simulink model "Target_Control_System"  (R2021b)
settings: Solver=FixedStepDiscrete  StartTime=0.0  StopTime=5  RelTol=1e-3
PreLoadFcn:
  | RTWConfigurationCB('preloadfcn', bdroot);
PostLoadFcn:
  | load('configuration/data_struct.mat');
  | load('configuration/fluxMaps_propMotor.mat');
  | load('configuration/parameterInit_PROP.mat');
  | load('configuration/parameterInit_PUMP.mat');
  | load('configuration/parameterInit_PITCH.mat');
  | load('configuration/parameterInit_TILT.mat');
  | %load('configuration/base_workspace_signal_definition.mat');
  | %load('resolvedatastores_to_baseworkspace_for_faster_simulation.mat');
model workspace (MAT data in the model file):
  SIMULATION_OPTIONS : Simulink.Parameter (value not decoded)
  TARGET_CODE_GEN : Simulink.Parameter (value not decoded)
  TCS_SAMPLE_FREQ_HZ : Simulink.Parameter (value not decoded)
symbols that are objects in the model workspace (value not decoded): TARGET_CODE_GEN, TCS_SAMPLE_FREQ_HZ
undefined symbols (not defined in the file): A_DQ_REF_LPF_INIT__PITCH, A_DQ_REF_LPF_INIT__PROP, A_DQ_REF_LPF_INIT__PUMP, A_DQ_REF_LPF_INIT__TILT, A_OBSERVER_CONFIDENCE_INIT__PITCH, A_OBSERVER_CONFIDENCE_INIT__PROP, A_OBSERVER_CONFIDENCE_INIT__PUMP, A_OBSERVER_CONFIDENCE_INIT__TILT, ACTUATOR_MAX_ANGLE_TRIP__PITCH, ACTUATOR_MIN_ANGLE_TRIP__PITCH, ACTUATOR_POS_SENSOR_INV_DIRECTION__PITCH, ACTUATOR_POS_SENSOR_INV_DIRECTION__TILT, ACTUATOR_POS_SENSOR_OFFSET__PITCH, ACTUATOR_POS_SENSOR_OFFSET__TILT, ADC_scaler1_baseaddr_TILT, ADC_SCALER_FLOAT_TO_FIXPOINT_EXPANSION, ANGLE_ELEC_FROM_SENSOR_OFFSET_INIT__PITCH, ANGLE_ELEC_FROM_SENSOR_OFFSET_INIT__PROP, ANGLE_ELEC_FROM_SENSOR_OFFSET_INIT__PUMP, ANGLE_ELEC_FROM_SENSOR_OFFSET_INIT__TILT, AUTO_CLEAR_FAULTS_ENABLED__PITCH, AUTO_CLEAR_FAULTS_ENABLED__PROP, AUTO_CLEAR_FAULTS_ENABLED__PUMP, AUTO_CLEAR_FAULTS_ENABLED__TILT, AUTO_CLEAR_FAULTS_WAIT_TICKS__PITCH, AUTO_CLEAR_FAULTS_WAIT_TICKS__PROP, AUTO_CLEAR_FAULTS_WAIT_TICKS__PUMP, AUTO_CLEAR_FAULTS_WAIT_TICKS__TILT, AUTO_I_ZERO_IDLE_TICKS__PITCH, AUTO_I_ZERO_IDLE_TICKS__PROP, AUTO_I_ZERO_IDLE_TICKS__PUMP, AUTO_I_ZERO_IDLE_TICKS__TILT, AUTO_I_ZERO_OFFSET_IDC_THRESHOLD__PITCH, AUTO_I_ZERO_OFFSET_IDC_THRESHOLD__PROP, AUTO_I_ZERO_OFFSET_IDC_THRESHOLD__PUMP, AUTO_I_ZERO_OFFSET_IDC_THRESHOLD__TILT, AUTO_I_ZERO_OFFSET_IPH_THRESHOLD__PITCH, AUTO_I_ZERO_OFFSET_IPH_THRESHOLD__PROP, AUTO_I_ZERO_OFFSET_IPH_THRESHOLD__PUMP, AUTO_I_ZERO_OFFSET_IPH_THRESHOLD__TILT, AUTO_SENSORLESS_SWITCHOVER_DISABLE_OMEGA, AUTO_SENSORLESS_SWITCHOVER_ENABLE_OMEGA, AUTO_SENSORLESS_SWITCHOVER_MIN_CONFIDENCE, AUXILIARY_PROTECTION_UNIT_BASEADDR__TILT, blanking_max_error_omega_INIT_PITCH, blanking_max_error_omega_INIT_TILT, blanking_max_error_position_INIT_PITCH, blanking_max_error_position_INIT_TILT, BRUTE_START_I_Q_REF_RAMP_SPEED__PITCH, BRUTE_START_I_Q_REF_RAMP_SPEED__PROP, BRUTE_START_I_Q_REF_RAMP_SPEED__PUMP, BRUTE_START_I_Q_REF_RAMP_SPEED__TILT, CONTROL_LOOP_DT_INIT__PITCH, CONTROL_LOOP_DT_INIT__PROP, CONTROL_LOOP_DT_INIT__PUMP, CONTROL_LOOP_DT_INIT__TILT, CORRECTION_FILTER_SCALE__PITCH, CORRECTION_FILTER_SCALE__PROP, CORRECTION_FILTER_SCALE__PUMP, CORRECTION_FILTER_SCALE__TILT ... (+458)
libraries: simulink x178, Reusables_Lib x24
(part 27 of 47)

== system Target_Control_System/Target_Control_System/InterruptFunction/tiltMotor_isrTask/pwmGeneration/Subsystem/Calculate Duty Cycles ==
  fUaRef : Inport
  fUbRef : Inport  Port=2
  fUcRef : Inport  Port=3
  fMaximumDuty : Inport  Port=4
  fHalfPositiveDuty : Inport  Port=5
  fPwmPeriodTicksFloat : Inport  Port=6
  Constant1 : Constant  Value=0.5  OutDataTypeStr=single  SampleTime=-1
  Constant11 : Constant  Value=-1  SampleTime=-1
  Constant4 : Constant  Value=0.5  OutDataTypeStr=single  SampleTime=-1
  Constant6 : Constant  Value=0.5  OutDataTypeStr=single  SampleTime=-1
  Data Type Conversion : DataTypeConversion  OutDataTypeStr=uint32
  Data Type Conversion1 : DataTypeConversion  OutDataTypeStr=uint32
  Data Type Conversion2 : DataTypeConversion  OutDataTypeStr=uint32
  Product{1,6..10} (6 alike) : Product
  Saturation Dynamic : simulink/Discontinuities/Saturation Dynamic  OutMin=[]  OutMax=[]  OutDataTypeStr=Inherit: Same as second input  OutDataType=fixdt(1, 16)  OutScaling=2^-10  DoSatur=off
  Saturation Dynamic1 : simulink/Discontinuities/Saturation Dynamic  OutMin=[]  OutMax=[]  OutDataTypeStr=Inherit: Same as second input  OutDataType=fixdt(1, 16)  OutScaling=2^-10  DoSatur=off
  Saturation Dynamic2 : simulink/Discontinuities/Saturation Dynamic  OutMin=[]  OutMax=[]  OutDataTypeStr=Inherit: Same as second input  OutDataType=fixdt(1, 16)  OutScaling=2^-10  DoSatur=off
  Sum1 : Sum  Inputs=|++  OutDataTypeStr=single
  Sum4 : Sum  Inputs=|++  OutDataTypeStr=single
  Sum5 : Sum  Inputs=|++  OutDataTypeStr=single
  uiPwmDutyTicksA : Outport
  uiPwmDutyTicksB : Outport  Port=2
  uiPwmDutyTicksC : Outport  Port=3
  wires:
  Data Type Conversion2/1 -> uiPwmDutyTicksC/1
  Data Type Conversion1/1 -> uiPwmDutyTicksB/1
  Data Type Conversion/1 -> uiPwmDutyTicksA/1
  fMaximumDuty/1 -> Saturation Dynamic/1, Saturation Dynamic1/1, Saturation Dynamic2/1
  fHalfPositiveDuty/1 -> Product1/2, Product7/2, Product6/2
  fPwmPeriodTicksFloat/1 -> Product10/2, Product9/2, Product8/2
  Constant1/1 -> Sum1/2
  fUbRef/1 -> Saturation Dynamic1/2
  fUcRef/1 -> Saturation Dynamic2/2
  fUaRef/1 -> Saturation Dynamic/2
  Sum1/1 -> Product8/1
  Product9/1 -> Data Type Conversion1/1
  Constant6/1 -> Sum5/2
  Saturation Dynamic/1 -> Product1/1
  Product7/1 -> Sum5/1
  Sum5/1 -> Product10/1
  Constant4/1 -> Sum4/2
  Product1/1 -> Sum1/1
  Product6/1 -> Sum4/1
  Constant11/1 -> Saturation Dynamic/3, Saturation Dynamic1/3, Saturation Dynamic2/3
  Sum4/1 -> Product9/1
  Product8/1 -> Data Type Conversion/1
  Saturation Dynamic2/1 -> Product7/1
  Saturation Dynamic1/1 -> Product6/1
  Product10/1 -> Data Type Conversion2/1

== system Target_Control_System/Target_Control_System/InterruptFunction/tiltMotor_isrTask/pwmGeneration/Subsystem/Zero sequence injection ==
  U_abc : Inport
  Demux : Demux  Outputs=3
  Gain4 : Gain  Gain=0.5
  Max : MinMax  Function=max  Inputs=3
  Max1 : MinMax  Inputs=3
  Sum6 : Sum  OutDataTypeStr=single
  Sum7 : Sum  Inputs=|+-  OutDataTypeStr=single
  Sum8 : Sum  Inputs=|+-  OutDataTypeStr=single
  Sum9 : Sum  Inputs=|+-  OutDataTypeStr=single
  fUaRef : Outport
  fUbRef : Outport  Port=2
  fUcRef : Outport  Port=3
  wires:
  U_abc/1 -> Demux/1
  Demux/3 -> Max1/3, Max/3, Sum9/1  "Uc"
  Max/1 -> Sum6/1
  Sum9/1 -> fUcRef/1  "fUcRef"
  Sum7/1 -> fUaRef/1  "fUaRef"
  Gain4/1 -> Sum7/2, Sum8/2, Sum9/2  "fUOffCenter"
  Demux/2 -> Max1/1, Max/2, Sum8/1  "Ub"
  Sum8/1 -> fUbRef/1  "fUbRef"
  Max1/1 -> Sum6/2
  Sum6/1 -> Gain4/1  "Umax+Umin"
  Demux/1 -> Sum7/1, Max/1, Max1/2  "Ua"

== system Target_Control_System/Target_Control_System/InterruptFunction/tiltMotor_setPwm/ModelSourceFPGATilt/IncludeCustomCode/System Update ==

== system Target_Control_System/Target_Control_System/MainLoop/pitchMotor_mainLoop/Decimation gate for 10 Hz Pitch/Function-Call Subsystem/Dynamic_current_limiting_pitch ==
  Constant5 : Constant  Value=0  OutDataTypeStr=single  SampleTime=-1
  Data Store Read2 : DataStoreRead  DataStoreName=oPitch  DataStoreElements=oPitch.oMot_.oParam_.fDynILimIntegratorLeakageFactor_  IndexOptions=Index vector (dialog)  Indices=1  OutputSizes=1
  Enabled Subsystem : Subsystem  TreatAsAtomicUnit=on
  GreaterThan : RelationalOperator  Operator=>  OutDataTypeStr=boolean  RndMeth=Simplest
  wires:
  GreaterThan/1 -> Enabled Subsystem/Enable
  Constant5/1 -> GreaterThan/2
  Data Store Read2/1 -> GreaterThan/1

== system Target_Control_System/Target_Control_System/MainLoop/pitchMotor_mainLoop/Decimation gate for 200 Hz Pitch/Function-Call Subsystem/Check zero current if inverter off ==
  function : TriggerPort  TriggerType=function-call  VariantControl=Variant
  AND : Logic  Inputs=3  AllPortsSameDT=off  OutDataTypeStr=boolean
  Constant : Constant  Value=200  OutDataTypeStr=uint32  SampleTime=-1
  Constant1 : Constant  Value=99  OutDataTypeStr=uint32  SampleTime=-1
  Constant2 : Constant  Value=0  OutDataTypeStr=uint32  SampleTime=-1
  Data Store Read1 : DataStoreRead  DataStoreName=oPitch  DataStoreElements=oPitch.oMot_.oState_.uiDriveState_  IndexOptions=Index vector (dialog)  Indices=1  OutputSizes=1
  Data Store Read2 : DataStoreRead  DataStoreName=oPitch  DataStoreElements=oPitch.oMot_.oState_.uiCurrentOffsetNullingPerformed_  IndexOptions=Index vector (dialog)  Indices=1  OutputSizes=1
  Enabled Subsystem : Subsystem  TreatAsAtomicUnit=on
  GreaterThan : RelationalOperator  Operator=>  OutDataTypeStr=boolean  RndMeth=Simplest
  GreaterThan1 : RelationalOperator  Operator=>  OutDataTypeStr=boolean  RndMeth=Simplest
  Less Than : RelationalOperator  Operator=<  OutDataTypeStr=boolean  RndMeth=Simplest
  wires:
  AND/1 -> Enabled Subsystem/Enable
  GreaterThan1/1 -> AND/3
  Constant2/1 -> GreaterThan1/2
  Data Store Read2/1 -> GreaterThan1/1
  Less Than/1 -> AND/2
  GreaterThan/1 -> AND/1
  Constant1/1 -> GreaterThan/2
  Constant/1 -> Less Than/2
  Data Store Read1/1 -> GreaterThan/1, Less Than/1

== system Target_Control_System/Target_Control_System/MainLoop/pitchMotor_mainLoop/Decimation gate for 200 Hz Pitch/Function-Call Subsystem/Current control inactive ==
  function : TriggerPort  TriggerType=function-call  VariantControl=Variant
  Constant : Constant  Value=0  OutDataTypeStr=uint32  SampleTime=-1
  Data Store Read : DataStoreRead  DataStoreName=oPitch  DataStoreElements=oPitch.oMot_.oOut_.uiCurrentControllerActive_  IndexOptions=Index vector (dialog)  Indices=1  OutputSizes=1
  Enabled Subsystem : Subsystem  TreatAsAtomicUnit=on
  GreaterThan : RelationalOperator  Operator=>  OutDataTypeStr=boolean  RndMeth=Simplest
  NOT : Logic  Operator=NOT  IconShape=distinctive  AllPortsSameDT=off  OutDataTypeStr=boolean
  wires:
  NOT/1 -> Enabled Subsystem/Enable
  GreaterThan/1 -> NOT/1
  Constant/1 -> GreaterThan/2
  Data Store Read/1 -> GreaterThan/1

== system Target_Control_System/Target_Control_System/MainLoop/pitchMotor_mainLoop/Decimation gate for 200 Hz Pitch/Function-Call Subsystem/Current offset nulling ==
  note: Try to perform current sensor offset nulling at least once as soon as possible:
      | (Subsequent nulling steps are performed only once the drive has been idle for a while)
  function : TriggerPort  TriggerType=function-call  VariantControl=Variant
  Constant2 : Constant  Value=0  OutDataTypeStr=uint32  SampleTime=-1
  Data Store Read2 : DataStoreRead  DataStoreName=oPitch  DataStoreElements=oPitch.oMot_.oState_.uiCurrentOffsetNullingPerformed_  IndexOptions=Index vector (dialog)  Indices=1  OutputSizes=1
  GreaterThan1 : RelationalOperator  Operator=>  OutDataTypeStr=boolean  RndMeth=Simplest
  NOT : Logic  Operator=NOT  IconShape=distinctive  AllPortsSameDT=off  OutDataTypeStr=boolean
  initiateOffsetNulling(&oPitch) : Subsystem  TreatAsAtomicUnit=on
  wires:
  NOT/1 -> initiateOffsetNulling(&oPitch)/Enable
  GreaterThan1/1 -> NOT/1
  Constant2/1 -> GreaterThan1/2
  Data Store Read2/1 -> GreaterThan1/1

== system Target_Control_System/Target_Control_System/MainLoop/pitchMotor_mainLoop/Decimation gate for 200 Hz Pitch/Function-Call Subsystem/DClink_overCurrentProtection ==
  function : TriggerPort  TriggerType=function-call  VariantControl=Variant
  Chart : Stateflow chart  TreatAsAtomicUnit=on

== system Target_Control_System/Target_Control_System/MainLoop/pitchMotor_mainLoop/Decimation gate for 200 Hz Pitch/Function-Call Subsystem/Forced current injection for broken input sensors ==
  function : TriggerPort  TriggerType=function-call  VariantControl=Variant
  Constant : Constant  Value=226  OutDataTypeStr=uint32  SampleTime=-1
  Constant1 : Constant  Value=227  OutDataTypeStr=uint32  SampleTime=-1
  Constant2 : Constant  Value=228  OutDataTypeStr=uint32  SampleTime=-1
  Data Store Read : DataStoreRead  DataStoreName=oPitch  DataStoreElements=oPitch.oMot_.oState_.uiDriveState_  IndexOptions=Index vector (dialog)  Indices=1  OutputSizes=1
  Enabled Subsystem : Subsystem  TreatAsAtomicUnit=on
  Equal : RelationalOperator  Operator===  OutDataTypeStr=boolean  RndMeth=Simplest
  Equal1 : RelationalOperator  Operator===  OutDataTypeStr=boolean  RndMeth=Simplest
  Equal2 : RelationalOperator  Operator===  OutDataTypeStr=boolean  RndMeth=Simplest
  OR : Logic  Operator=OR  Inputs=3  AllPortsSameDT=off  OutDataTypeStr=boolean
  wires:
  OR/1 -> Enabled Subsystem/Enable
  Equal2/1 -> OR/3
  Equal/1 -> OR/1
  Equal1/1 -> OR/2
  Constant2/1 -> Equal2/2
  Constant1/1 -> Equal1/2
  Constant/1 -> Equal/2
  Data Store Read/1 -> Equal/1, Equal1/1, Equal2/1

== system Target_Control_System/Target_Control_System/MainLoop/pitchMotor_mainLoop/Decimation gate for 200 Hz Pitch/Function-Call Subsystem/Idle controller ==
  function : TriggerPort  TriggerType=function-call  VariantControl=Variant
  Constant : Constant  Value=211  OutDataTypeStr=uint32  SampleTime=-1
  Constant1 : Constant  Value=212  OutDataTypeStr=uint32  SampleTime=-1
  Data Store Read : DataStoreRead  DataStoreName=oPitch  DataStoreElements=oPitch.oMot_.oState_.uiDriveState_  IndexOptions=Index vector (dialog)  Indices=1  OutputSizes=1
  Equal : RelationalOperator  Operator===  OutDataTypeStr=boolean  RndMeth=Simplest
  Equal1 : RelationalOperator  Operator===  OutDataTypeStr=boolean  RndMeth=Simplest
  Forced angle : Subsystem  TreatAsAtomicUnit=on
  NOT : Logic  Operator=NOT  IconShape=distinctive  AllPortsSameDT=off  OutDataTypeStr=boolean
  Not forced angle : Subsystem  TreatAsAtomicUnit=on
  OR : Logic  Operator=OR  AllPortsSameDT=off  OutDataTypeStr=boolean
  wires:
  NOT/1 -> Not forced angle/Enable
  OR/1 -> NOT/1, Forced angle/Enable
  Equal1/1 -> OR/2
  Equal/1 -> OR/1
  Constant1/1 -> Equal1/2
  Data Store Read/1 -> Equal/1, Equal1/1
  Constant/1 -> Equal/2

== system Target_Control_System/Target_Control_System/MainLoop/pitchMotor_mainLoop/Decimation gate for 200 Hz Pitch/Function-Call Subsystem/Position control checks ==
  function : TriggerPort  TriggerType=function-call  VariantControl=Variant
  Constant : Constant  Value=0  OutDataTypeStr=int32  SampleTime=-1
  Data Store Read : DataStoreRead  DataStoreName=oPitch  DataStoreElements=oPitch.oMot_.oState_.oPosSensor_.iPosControlEnabled_  IndexOptions=Index vector (dialog)  Indices=1  OutputSizes=1
  GreaterThan : RelationalOperator  Operator=>  OutDataTypeStr=boolean  RndMeth=Simplest
  NOT : Logic  Operator=NOT  IconShape=distinctive  AllPortsSameDT=off  OutDataTypeStr=boolean
  NOT position control mode : Subsystem  TreatAsAtomicUnit=on
  Position control mode : Subsystem  TreatAsAtomicUnit=on
  Scope : Scope
  wires:
  NOT/1 -> NOT position control mode/Enable
  Constant/1 -> GreaterThan/2
  Data Store Read/1 -> GreaterThan/1
  GreaterThan/1 -> Position control mode/Enable, NOT/1, Scope/1

== system Target_Control_System/Target_Control_System/MainLoop/pitchMotor_mainLoop/Decimation gate for 5000 Hz Pitch/motorTaskProcessExternalSetpoints(&oPitch)/hot_standby ==
  hot_standby : TriggerPort  TriggerType=function-call  VariantControl=Variant
  AND5 : Logic  Operator=OR  AllPortsSameDT=off  OutDataTypeStr=boolean
  Data Store Read85 : DataStoreRead  DataStoreName=oPitch  DataStoreElements=oPitch.oMot_.oState_.uiDriveState_  IndexOptions=Index vector (dialog)  Indices=1  OutputSizes=1
  Equal1 : RelationalOperator  Operator===  OutDataTypeStr=boolean  RndMeth=Simplest
  Equal13 : RelationalOperator  Operator===  OutDataTypeStr=boolean  RndMeth=Simplest
  Subsystem : Subsystem
  const1 : Constant  Value=235  OutDataTypeStr=uint32  SampleTime=-1
  const2 : Constant  Value=236  OutDataTypeStr=uint32  SampleTime=-1
  wires:
  const2/1 -> Equal1/2
  const1/1 -> Equal13/2
  Data Store Read85/1 -> Equal13/1, Equal1/1
  Equal1/1 -> AND5/2
  AND5/1 -> Subsystem/Enable
  Equal13/1 -> AND5/1

== system Target_Control_System/Target_Control_System/MainLoop/pitchMotor_mainLoop/Decimation gate for 5000 Hz Pitch/motorTaskProcessExternalSetpoints(&oPitch)/passive_holding_mode ==
  passive_holding_mode : TriggerPort  TriggerType=function-call  VariantControl=Variant
  AND5 : Logic  Operator=OR  Inputs=3  AllPortsSameDT=off  OutDataTypeStr=boolean
  Data Store Read85 : DataStoreRead  DataStoreName=oPitch  DataStoreElements=oPitch.oMot_.oState_.uiDriveState_  IndexOptions=Index vector (dialog)  Indices=1  OutputSizes=1
  Equal1 : RelationalOperator  Operator===  OutDataTypeStr=boolean  RndMeth=Simplest
  Equal13 : RelationalOperator  Operator===  OutDataTypeStr=boolean  RndMeth=Simplest
  Equal2 : RelationalOperator  Operator===  OutDataTypeStr=boolean  RndMeth=Simplest
  Subsystem : Subsystem
  const1 : Constant  Value=226  OutDataTypeStr=uint32  SampleTime=-1
  const2 : Constant  Value=227  OutDataTypeStr=uint32  SampleTime=-1
  const3 : Constant  Value=228  OutDataTypeStr=uint32  SampleTime=-1
  wires:
  const3/1 -> Equal2/2
  const2/1 -> Equal1/2
  const1/1 -> Equal13/2
  Data Store Read85/1 -> Equal13/1, Equal1/1, Equal2/1
  Equal1/1 -> AND5/2
  Equal2/1 -> AND5/3
  AND5/1 -> Subsystem/Enable
  Equal13/1 -> AND5/1

== system Target_Control_System/Target_Control_System/MainLoop/pitchMotor_mainLoop/Decimation gate for 5000 Hz Pitch/motorTaskProcessExternalSetpoints(&oPitch)/set_target ==
  note: // Position target
  note: // Speed target
  note: Iq current (that is, torque target)
  note: // Do Id
  note: // (Iq is controlled by the forced angle sequencer)
  note: // Forced angle start regime, ensure that Id is zero
  set_target : TriggerPort  TriggerType=function-call  VariantControl=Variant
  AND1 : Logic  AllPortsSameDT=off  OutDataTypeStr=boolean
  AND5 : Logic  Inputs=3  AllPortsSameDT=off  OutDataTypeStr=boolean
  Data Store Read85 : DataStoreRead  DataStoreName=oPitch  DataStoreElements=oPitch.oMot_.oState_.uiDriveState_  IndexOptions=Index vector (dialog)  Indices=1  OutputSizes=1
  Equal1 : RelationalOperator  OutDataTypeStr=boolean  RndMeth=Simplest
  Equal13 : RelationalOperator  Operator=~=  OutDataTypeStr=boolean  RndMeth=Simplest
  Equal14 : RelationalOperator  Operator=~=  OutDataTypeStr=boolean  RndMeth=Simplest
  Equal2 : RelationalOperator  Operator=<=  OutDataTypeStr=boolean  RndMeth=Simplest
  Id_target : Subsystem
  Id_zero_for_forced_angle : Subsystem
  Iq_target : Subsystem
  NOT : Logic  Operator=NOT  AllPortsSameDT=off  OutDataTypeStr=boolean
  NOT1 : Logic  Operator=NOT  AllPortsSameDT=off  OutDataTypeStr=boolean
  const1 : Constant  Value=245  OutDataTypeStr=uint32  SampleTime=-1
  const17 : Constant  Value=211  OutDataTypeStr=uint32  SampleTime=-1
  const18 : Constant  Value=212  OutDataTypeStr=uint32  SampleTime=-1
  const2 : Constant  Value=254  OutDataTypeStr=uint32  SampleTime=-1
  position_target : Subsystem
  speed_target : Subsystem
  wires:
  NOT1/1 -> Id_zero_for_forced_angle/Enable
  AND5/1 -> NOT1/1, position_target/Enable, Iq_target/Enable, Id_target/Enable, speed_target/Enable
  Equal13/1 -> AND5/1
  Equal1/1 -> AND1/1
  const18/1 -> Equal14/2
  Equal2/1 -> AND1/2
  AND1/1 -> NOT/1
  const17/1 -> Equal13/1
  Data Store Read85/1 -> Equal2/1, Equal1/1, Equal14/1, Equal13/2
  const2/1 -> Equal2/2
  NOT/1 -> AND5/3
  const1/1 -> Equal1/2
  Equal14/1 -> AND5/2

== system Target_Control_System/Target_Control_System/MainLoop/pitchMotor_mainLoop/mainTask_pitch/PWM for Simulation/Subsystem ==
  Enable : EnablePort
  Bus Creator1 : BusCreator  Inputs=3
  Data Store Read7 : DataStoreRead  DataStoreName=oPitch  DataStoreElements=oPitch.oIsr_.oOut_.uiPwmDutyTicksA_  IndexOptions=Index vector (dialog)  Indices=1  OutputSizes=1
  Data Store Read8 : DataStoreRead  DataStoreName=oPitch  DataStoreElements=oPitch.oIsr_.oOut_.uiPwmDutyTicksB_  IndexOptions=Index vector (dialog)  Indices=1  OutputSizes=1
  Data Store Read9 : DataStoreRead  DataStoreName=oPitch  DataStoreElements=oPitch.oIsr_.oOut_.uiPwmDutyTicksC_  IndexOptions=Index vector (dialog)  Indices=1  OutputSizes=1
  pitchMotor_PWMticks : Outport
  wires:
  Data Store Read8/1 -> Bus Creator1/2  "Bticks"
  Bus Creator1/1 -> pitchMotor_PWMticks/1
  Data Store Read9/1 -> Bus Creator1/3  "Cticks"
  Data Store Read7/1 -> Bus Creator1/1  "Aticks"

== system Target_Control_System/Target_Control_System/MainLoop/pitchMotor_mainLoop/mainTask_pitch/PWM for Simulation/Subsystem1 ==
  Enable : EnablePort
  Data Store Read6 : DataStoreRead  DataStoreName=oPitch  DataStoreElements=oPitch.oMot_.oOut_.uiPwmRequestFromMain_  IndexOptions=Index vector (dialog)  Indices=1  OutputSizes=1
  Scope : Scope
  Subsystem : Subsystem
  pitchMotor_PWMticks : Outport
  wires:
  Data Store Read6/1 -> Subsystem/Enable, Scope/1
  Subsystem/1(pitchMotor_PWMticks) -> pitchMotor_PWMticks/1

== system Target_Control_System/Target_Control_System/MainLoop/pitchMotor_mainLoop/mainTask_pitch/Variant Subsystem/Target_Code_Gen_0 ==
  Function-Call Generator : simulink/Ports & Subsystems/Function-Call Generator  sample_time=-1  numberOfIterations=1  DisallowWideOutput=off
  Output : Outport
  wires:
  Function-Call Generator/1 -> Output/1

== system Target_Control_System/Target_Control_System/MainLoop/pitchMotor_mainLoop/mainTask_pitch/Variant Subsystem/Target_Code_Gen_1 ==
  Data Store Read4 : DataStoreRead  DataStoreName=oPitch  DataStoreElements=oPitch.oMot_.oIn_.uiDataFromIsrToMainUpdated_  IndexOptions=Index vector (dialog)  Indices=1  OutputSizes=1
  Triggered Subsystem : Subsystem  TreatAsAtomicUnit=on
  Output : Outport
  wires:
  Triggered Subsystem/1(Output) -> Output/1
  Data Store Read4/1 -> Triggered Subsystem/Trigger

== system Target_Control_System/Target_Control_System/MainLoop/pitchMotor_mainLoop/mainTask_pitch/motorTaskMainFastStep()/Automatic switching to sensorless - Pitch ==
  autoSwitchToSensorless : TriggerPort  TriggerType=function-call  VariantControl=Variant
  Automatic switching to sensorless : Subsystem  TreatAsAtomicUnit=on
  Constant : Constant  Value=0  SampleTime=-1
  Data Store Read4 : DataStoreRead  DataStoreName=oPitch  DataStoreElements=oPitch.oMot_.oParam_.uiSensorlessSwitchoverMode_  IndexOptions=Index vector (dialog)  Indices=1  OutputSizes=1
  GreaterThan : RelationalOperator  Operator=>  OutDataTypeStr=boolean  RndMeth=Simplest
  wires:
  Constant/1 -> GreaterThan/2
  GreaterThan/1 -> Automatic switching to sensorless/Enable
  Data Store Read4/1 -> GreaterThan/1

== system Target_Control_System/Target_Control_System/MainLoop/pitchMotor_mainLoop/mainTask_pitch/motorTaskMainFastStep()/Control Loops - Pitch ==
  note: // Ramp position setpoint
  note: // Blend in the idle controller's contribution (don't add; disturbs Torque/Amp relation).
      | // Take the max of both, but only if the idle controller is active)
  note: // Static current limiting only
  note: // Ramp angle compensation value for smoothing of forced to closed loop operation
      |  // It always ramps to zero.
  note: // Ramp Id, also include a fixed fraction of Iq (happens in the interupt)
  note: // Feed-forward of speed reference derivative into torque
      | // --- Would go here if needed --- (Blend the ramp generator ddt output into Iq ref)
  note: // The greater than 0 is needed to allow regen braking when the speed is high enough
  note: // no feedforward in forced angle, because the speed estimate may be garbage
  note: // Ramp speed setpoint
  note: // // Feed forward from position reference to speed setpoint
  controlLoops : TriggerPort  TriggerType=function-call  VariantControl=Variant
  AND : Logic  AllPortsSameDT=off  OutDataTypeStr=boolean
  Constant : Constant  Value=0.001  OutDataTypeStr=single  SampleTime=-1
  Constant1 : Constant  Value=0  SampleTime=-1
  Constant11 : Constant  Value=ISR_FREQ_KHZ__PITCH  OutDataTypeStr=single  SampleTime=-1
  Constant12 : Constant  Value=CONTROL_LOOP_DT_INIT__PITCH  OutDataTypeStr=single  SampleTime=-1
  Constant13 : Constant  Value=0  OutDataTypeStr=uint32  SampleTime=-1
  Constant2 : Constant  Commented=on  Value=0  SampleTime=-1
  Constant5 : Constant  Commented=on  Value=0  OutDataTypeStr=single  SampleTime=-1
  Constant9 : Constant  Value=0  SampleTime=-1
  Data Store Read1 : DataStoreRead  Commented=on  DataStoreName=oPitch  DataStoreElements=oPitch.oMot_.oState_.oRampDataFluxMasterAngleOffset_.fSetpoint_  IndexOptions=Index vector (dialog)  Indices=1  OutputSizes=1
  Data Store Read10 : DataStoreRead  DataStoreName=oPitch  DataStoreElements=oPitch.oMot_.oParam_.fDynILimIntegratorLeakageFactor_  IndexOptions=Index vector (dialog)  Indices=1  OutputSizes=1
  Data Store Read12 : DataStoreRead  DataStoreName=oPitch  DataStoreElements=oPitch.oMot_.oState_.fIdleCtrlCurrent_  IndexOptions=Index vector (dialog)  Indices=1  OutputSizes=1
  Data Store Read14 : DataStoreRead  DataStoreName=oPitch  DataStoreElements=oPitch.oMot_.oParam_.fIqSetpointMax_  IndexOptions=Index vector (dialog)  Indices=1  OutputSizes=1
  Data Store Read15 : DataStoreRead  DataStoreName=oPitch  DataStoreElements=oPitch.oMot_.oState_.oRampDataIdRef_.oParam_.fTimestepS_  IndexOptions=Index vector (dialog)  Indices=1  OutputSizes=1
  Data Store Read16 : DataStoreRead  DataStoreName=oPitch  DataStoreElements=oPitch.oMot_.oState_.oRampDataIdRef_.oParam_.fUpslope_  IndexOptions=Index vector (dialog)  Indices=1  OutputSizes=1
  Data Store Read17 : DataStoreRead  DataStoreName=oPitch  DataStoreElements=oPitch.oMot_.oState_.oRampDataIdRef_.oParam_.fDownslope_  IndexOptions=Index vector (dialog)  Indices=1  OutputSizes=1
  Data Store Read18 : DataStoreRead  Commented=on  DataStoreName=oPitch  DataStoreElements=oPitch.oMot_.oOut_.uiForcedAngle_  IndexOptions=Index vector (dialog)  Indices=1  OutputSizes=1
  Data Store Read2 : DataStoreRead  DataStoreName=oPitch  DataStoreElements=oPitch.oMot_.oState_.oPosSensor_.iPosControlEnabled_  IndexOptions=Index vector (dialog)  Indices=1  OutputSizes=1
  Data Store Read23 : DataStoreRead  Commented=on  DataStoreName=oPitch  DataStoreElements=oPitch.oMot_.oState_.oRampDataFluxFeedforwardGain_.fRampOut_  IndexOptions=Index vector (dialog)  Indices=1  OutputSizes=1
  Data Store Read24 : DataStoreRead  Commented=on  DataStoreName=oPitch  DataStoreElements=oPitch.oMot_.oState_.oRampDataFluxMasterAngleOffset_.oParam_.fTimestepS_  IndexOptions=Index vector (dialog)  Indices=1  OutputSizes=1
  Data Store Read25 : DataStoreRead  Commented=on  DataStoreName=oPitch  DataStoreElements=oPitch.oMot_.oState_.oRampDataFluxMasterAngleOffset_.oParam_.fUpslope_  IndexOptions=Index vector (dialog)  Indices=1  OutputSizes=1
  Data Store Read26 : DataStoreRead  Commented=on  DataStoreName=oPitch  DataStoreElements=oPitch.oMot_.oState_.oRampDataFluxMasterAngleOffset_.oParam_.fDownslope_  IndexOptions=Index vector (dialog)  Indices=1  OutputSizes=1
  Data Store Read3 : DataStoreRead  DataStoreName=oPitch  DataStoreElements=oPitch.oMot_.oParam_.fPositionRefFfwdToOmega_  IndexOptions=Index vector (dialog)  Indices=1  OutputSizes=1
  Data Store Read5 : DataStoreRead  DataStoreName=oPitch  DataStoreElements=oPitch.oMot_.oState_.oRampDataOmegaERef_.fSetpoint_  IndexOptions=Index vector (dialog)  Indices=1  OutputSizes=1
  Data Store Read6 : DataStoreRead  DataStoreName=oPitch  DataStoreElements=oPitch.oMot_.oState_.oRampDataOmegaERef_.oParam_.fTimestepS_  IndexOptions=Index vector (dialog)  Indices=1  OutputSizes=1
  Data Store Read7 : DataStoreRead  DataStoreName=oPitch  DataStoreElements=oPitch.oMot_.oState_.oRampDataOmegaERef_.oParam_.fUpslope_  IndexOptions=Index vector (dialog)  Indices=1  OutputSizes=1
  Data Store Read71 : DataStoreRead  DataStoreName=oPitch  DataStoreElements=oPitch.oMot_.oState_.oRampDataIqRef_.oParam_.fTimestepS_  IndexOptions=Index vector (dialog)  Indices=1  OutputSizes=1
  Data Store Read73 : DataStoreRead  DataStoreName=oPitch  DataStoreElements=oPitch.oMot_.oState_.oRampDataIqRef_.oParam_.fUpslope_  IndexOptions=Index vector (dialog)  Indices=1  OutputSizes=1
  Data Store Read74 : DataStoreRead  DataStoreName=oPitch  DataStoreElements=oPitch.oMot_.oState_.fIqRefBeforeRamp_  IndexOptions=Index vector (dialog)  Indices=1  OutputSizes=1
  Data Store Read75 : DataStoreRead  Commented=on  DataStoreName=oPitch  DataStoreElements=oPitch.oMot_.oState_.oRampDataFluxMstrAngFrcd2clsdSmoothn_.oParam_.fUpslope_  IndexOptions=Index vector (dialog)  Indices=1  OutputSizes=1
  Data Store Read76 : DataStoreRead  DataStoreName=oPitch  DataStoreElements=oPitch.oMot_.oState_.oRampDataIqRef_.oParam_.fDownslope_  IndexOptions=Index vector (dialog)  Indices=1  OutputSizes=1
  Data Store Read78 : DataStoreRead  DataStoreName=oPitch  DataStoreElements=oPitch.oMot_.oState_.oRampDataPos_.oParam_.fUpslope_  IndexOptions=Index vector (dialog)  Indices=1  OutputSizes=1
  Data Store Read8 : DataStoreRead  DataStoreName=oPitch  DataStoreElements=oPitch.oMot_.oState_.uiSpeedControllerActive_  IndexOptions=Index vector (dialog)  Indices=1  OutputSizes=1
  Data Store Read80 : DataStoreRead  DataStoreName=oPitch  DataStoreElements=oPitch.oMot_.oState_.oRampDataPos_.oParam_.fDownslope_  IndexOptions=Index vector (dialog)  Indices=1  OutputSizes=1
  Data Store Read82 : DataStoreRead  DataStoreName=oPitch  DataStoreElements=oPitch.oMot_.oState_.oRampDataPos_.fSetpoint_  IndexOptions=Index vector (dialog)  Indices=1  OutputSizes=1
  Data Store Read89 : DataStoreRead  Commented=on  DataStoreName=oPitch  DataStoreElements=oPitch.oMot_.oState_.oRampDataFluxMstrAngFrcd2clsdSmoothn_.oParam_.fDownslope_  IndexOptions=Index vector (dialog)  Indices=1  OutputSizes=1
  Data Store Read9 : DataStoreRead  DataStoreName=oPitch  DataStoreElements=oPitch.oMot_.oState_.oRampDataOmegaERef_.oParam_.fDownslope_  IndexOptions=Index vector (dialog)  Indices=1  OutputSizes=1
  Data Store Read90 : DataStoreRead  Commented=on  DataStoreName=oPitch  DataStoreElements=oPitch.oMot_.oState_.oRampDataFluxMstrAngFrcd2clsdSmoothn_.oParam_.fTimestepS_  IndexOptions=Index vector (dialog)  Indices=1  OutputSizes=1
  Data Store Write1 : DataStoreWrite  Commented=on  DataStoreName=oPitch  DataStoreElements=oPitch.oMot_.oState_.oRampDataFluxMstrAngFrcd2clsdSmoothn_.fSetpoint_  IndexOptions=Index vector (dialog)  Indices=1  OutputSizes=1
  Data Store Write11 : DataStoreWrite  Commented=on  DataStoreName=oPitch  DataStoreElements=oPitch.oMot_.oState_.oRampDataFluxMasterAngleOffset_.fRampOut_  IndexOptions=Index vector (dialog)  Indices=1  OutputSizes=1
  Data Store Write12 : DataStoreWrite  Commented=on  DataStoreName=oPitch  DataStoreElements=oPitch.oMot_.oState_.oRampDataFluxMasterAngleOffset_.fRampOutDdt_  IndexOptions=Index vector (dialog)  Indices=1  OutputSizes=1
  Data Store Write13 : DataStoreWrite  Commented=on  DataStoreName=oPitch  DataStoreElements=oPitch.oMot_.oState_.oRampDataFluxMstrAngFrcd2clsdSmoothn_.fRampOut_  IndexOptions=Index vector (dialog)  Indices=1  OutputSizes=1
  Data Store Write15 : DataStoreWrite  Commented=on  DataStoreName=oPitch  DataStoreElements=oPitch.oMot_.oState_.oRampDataFluxMstrAngFrcd2clsdSmoothn_.fRampOutDdt_  IndexOptions=Index vector (dialog)  Indices=1  OutputSizes=1
  Data Store Write18 : DataStoreWrite  DataStoreName=oPitch  DataStoreElements=oPitch.oMot_.oState_.oRampDataIqRef_.fRampOut_  IndexOptions=Index vector (dialog)  Indices=1  OutputSizes=1
  Data Store Write2 : DataStoreWrite  DataStoreName=oPitch  DataStoreElements=oPitch.oMot_.oState_.oRampDataOmegaERef_.fRampOut_  IndexOptions=Index vector (dialog)  Indices=1  OutputSizes=1
  Data Store Write23 : DataStoreWrite  DataStoreName=oPitch  DataStoreElements=oPitch.oMot_.oState_.oRampDataPos_.fRampOut_  IndexOptions=Index vector (dialog)  Indices=1  OutputSizes=1
  Data Store Write26 : DataStoreWrite  DataStoreName=oPitch  DataStoreElements=oPitch.oMot_.oState_.oRampDataIqRef_.fRampOutDdt_  IndexOptions=Index vector (dialog)  Indices=1  OutputSizes=1
  Data Store Write27 : DataStoreWrite  DataStoreName=oPitch  DataStoreElements=oPitch.oMot_.oState_.oRampDataPos_.fRampOutDdt_  IndexOptions=Index vector (dialog)  Indices=1  OutputSizes=1
  Data Store Write3 : DataStoreWrite  DataStoreName=oPitch  DataStoreElements=oPitch.oMot_.oState_.oRampDataOmegaERef_.fRampOutDdt_  IndexOptions=Index vector (dialog)  Indices=1  OutputSizes=1
  Data Store Write4 : DataStoreWrite  DataStoreName=oPitch  DataStoreElements=oPitch.oMot_.oState_.oRampDataIqRef_.fSetpoint_  IndexOptions=Index vector (dialog)  Indices=1  OutputSizes=1
  Data Store Write5 : DataStoreWrite  DataStoreName=oPitch  DataStoreElements=oPitch.oMot_.oState_.oRampDataIdRef_.fSetpoint_  IndexOptions=Index vector (dialog)  Indices=1  OutputSizes=1
  Data Store Write7 : DataStoreWrite  DataStoreName=oPitch  DataStoreElements=oPitch.oMot_.oState_.oRampDataIdRef_.fRampOut_  IndexOptions=Index vector (dialog)  Indices=1  OutputSizes=1
  Data Store Write8 : DataStoreWrite  DataStoreName=oPitch  DataStoreElements=oPitch.oMot_.oState_.oRampDataIdRef_.fRampOutDdt_  IndexOptions=Index vector (dialog)  Indices=1  OutputSizes=1
  Data Store Write9 : DataStoreWrite  Commented=on  DataStoreName=oPitch  DataStoreElements=oPitch.oMot_.oState_.oRampDataFluxFeedforwardGain_.fRampOut_  IndexOptions=Index vector (dialog)  Indices=1  OutputSizes=1
  Divide : Product  Inputs=**
  Dynamic Current Limiting Pitch : Subsystem  Commented=on  TreatAsAtomicUnit=on
  Flux Weakening - Pitch : Subsystem
  Gain : Gain  Gain=-1
  GreaterThan{,1..3} (4 alike) : RelationalOperator  Operator=>  OutDataTypeStr=boolean  RndMeth=Simplest
  GreaterThan4 : RelationalOperator  Commented=on  Operator=>  OutDataTypeStr=boolean  RndMeth=Simplest
  Max1 : MinMax  Function=max  Inputs=2
  Min : MinMax  Inputs=2
  NOT : Logic  Commented=on  Operator=NOT  AllPortsSameDT=off  OutDataTypeStr=boolean
  Position Controller Pitch : Subsystem  TreatAsAtomicUnit=on
  Ramp Flux Feedforward : Subsystem  Commented=on  TreatAsAtomicUnit=on
  Speed Controller Pitch : Subsystem  TreatAsAtomicUnit=on
  Sum : Sum  Inputs=|++
  Switch : Switch  Criteria=u2 > Threshold
  Switch1 : Switch  Criteria=u2 > Threshold
  Switch2 : Switch  Criteria=u2 > Threshold
  Switch4 : Switch  Commented=on  Criteria=u2 > Threshold
  Unit Delay3 : UnitDelay  SampleTime=-1  HasFrameUpgradeWarning=on
  Zero11 : Constant  Commented=on  Value=0  OutDataTypeStr=single  SampleTime=-1
  pp_pitch : Gain  Gain=POLE_PAIRS_INIT__PITCH  ParamDataTypeStr=single
  rampStep(oRampDataFluxMasterAngleOffset)_pitch : Reusables_Lib/rampStep_  Commented=on  SystemSampleTime=-1  VariantActivationTime=update diagram  Latency=0  AutoFrameSizeCalculation=off
  rampStep(oRampDataFluxMstrAngFrcd2clsdSmoothn)_pitch : Reusables_Lib/rampStep_  Commented=on  SystemSampleTime=-1  VariantActivationTime=update diagram  Latency=0  AutoFrameSizeCalculation=off
  rampStep(oRampDataIdRef)_pitch : Reusables_Lib/rampStep_  SystemSampleTime=-1  VariantActivationTime=update diagram  Latency=0  AutoFrameSizeCalculation=off
  rampStep(oRampDataIqRef)_pitch : Reusables_Lib/rampStep_  SystemSampleTime=-1  VariantActivationTime=update diagram  Latency=0  AutoFrameSizeCalculation=off
  rampStep(oRampDataOmegaERef)_pitch : Reusables_Lib/rampStep_  SystemSampleTime=-1  VariantActivationTime=update diagram  Latency=0  AutoFrameSizeCalculation=off
  rampStep(oRampDataPos) : Reusables_Lib/rampStep(oRampDataPos)  SystemSampleTime=-1  VariantActivationTime=update diagram  Latency=0  AutoFrameSizeCalculation=off
  to_CTRL_Hz : Gain  Gain=2*1000  ParamDataTypeStr=single  OutDataTypeStr=single
  wires:
  rampStep(oRampDataOmegaERef)_pitch/2 -> Data Store Write3/1
  rampStep(oRampDataIqRef)_pitch/2 -> Data Store Write26/1
  rampStep(oRampDataIqRef)_pitch/1 -> Data Store Write18/1
  rampStep(oRampDataIdRef)_pitch/1 -> Data Store Write7/1
  rampStep(oRampDataFluxMstrAngFrcd2clsdSmoothn)_pitch/2 -> Data Store Write15/1
  rampStep(oRampDataFluxMstrAngFrcd2clsdSmoothn)_pitch/1 -> Data Store Write13/1
  rampStep(oRampDataFluxMasterAngleOffset)_pitch/2 -> Data Store Write12/1
  Data Store Read7/1 -> rampStep(oRampDataOmegaERef)_pitch/2
  Data Store Read6/1 -> rampStep(oRampDataOmegaERef)_pitch/4
  Data Store Read24/1 -> rampStep(oRampDataFluxMasterAngleOffset)_pitch/4
  Data Store Read90/1 -> rampStep(oRampDataFluxMstrAngFrcd2clsdSmoothn)_pitch/4
  rampStep(oRampDataPos)/1 -> Data Store Write23/1, Unit Delay3/1, Position Controller Pitch/1(oRampDataPos_.fRampOut)
  Constant5/1 -> Switch4/1
  Constant11/1 -> to_CTRL_Hz/1
  pp_pitch/1 -> Divide/1
  Data Store Read12/1 -> Switch2/1, GreaterThan/1, GreaterThan1/1
  Data Store Read16/1 -> rampStep(oRampDataIdRef)_pitch/2
  Data Store Read80/1 -> rampStep(oRampDataPos)/4
  Data Store Read89/1 -> rampStep(oRampDataFluxMstrAngFrcd2clsdSmoothn)_pitch/3
  rampStep(oRampDataIdRef)_pitch/2 -> Data Store Write8/1
  Switch1/1 -> Switch2/3, GreaterThan1/2  "oRampDataIqRef_.fSetpoint"
  Min/1 -> Max1/1
  Data Store Read78/1 -> rampStep(oRampDataPos)/3
  Data Store Read74/1 -> Min/1
  rampStep(oRampDataOmegaERef)_pitch/1 -> Speed Controller Pitch/1(oRampDataOmegaERef_.fRampOut), Data Store Write2/1
  Switch4/1 -> Data Store Write9/1
  Data Store Read8/1 -> Speed Controller Pitch/Enable
  NOT/1 -> Ramp Flux Feedforward/Enable
  Flux Weakening - Pitch/1(oRampDataIdRef_.fSetpoint) -> Data Store Write5/1, rampStep(oRampDataIdRef)_pitch/1
  Data Store Read3/1 -> Divide/2
  GreaterThan4/1 -> NOT/1, Switch4/2
  Unit Delay3/1 -> rampStep(oRampDataPos)/2
  Constant9/1 -> GreaterThan2/2
  Data Store Read5/1 -> Switch/3
  rampStep(oRampDataFluxMasterAngleOffset)_pitch/1 -> Data Store Write11/1
  Data Store Read26/1 -> rampStep(oRampDataFluxMasterAngleOffset)_pitch/3
  Data Store Read14/1 -> Gain/1, Min/2
  GreaterThan3/1 -> Switch/2, Position Controller Pitch/Enable
  Constant2/1 -> GreaterThan4/2
  Data Store Read76/1 -> rampStep(oRampDataIqRef)_pitch/3
  Data Store Read15/1 -> rampStep(oRampDataIdRef)_pitch/4
  Zero11/1 -> rampStep(oRampDataFluxMstrAngFrcd2clsdSmoothn)_pitch/1, Data Store Write1/1
  Constant1/1 -> GreaterThan3/2
  Data Store Read71/1 -> rampStep(oRampDataIqRef)_pitch/4
  AND/1 -> Switch2/2
  Constant/1 -> GreaterThan/2
  Switch/1 -> Sum/2
  Data Store Read73/1 -> rampStep(oRampDataIqRef)_pitch/2
  GreaterThan/1 -> AND/1
  Constant13/1 -> Switch1/2
  Data Store Read1/1 -> rampStep(oRampDataFluxMasterAngleOffset)_pitch/1
  Max1/1 -> Switch1/3
  Switch2/1 -> Data Store Write4/1, rampStep(oRampDataIqRef)_pitch/1
  Position Controller Pitch/1(oRampDataOmegaERef_.fSetpoint) -> Switch/1
  GreaterThan1/1 -> AND/2
  Constant12/1 -> rampStep(oRampDataPos)/6
  Data Store Read9/1 -> rampStep(oRampDataOmegaERef)_pitch/3
  Data Store Read82/1 -> rampStep(oRampDataPos)/1
  Data Store Read75/1 -> rampStep(oRampDataFluxMstrAngFrcd2clsdSmoothn)_pitch/2
  rampStep(oRampDataPos)/2 -> Data Store Write27/1, pp_pitch/1
  Data Store Read2/1 -> GreaterThan3/1
  Sum/1 -> rampStep(oRampDataOmegaERef)_pitch/1
  Dynamic Current Limiting Pitch/1(oRampDataIqRef_.fSetpoint) -> Switch1/1
  Data Store Read23/1 -> Switch4/3
  to_CTRL_Hz/1 -> rampStep(oRampDataPos)/5
  Gain/1 -> Max1/2
  GreaterThan2/1 -> Dynamic Current Limiting Pitch/Enable
  Divide/1 -> Sum/1
  Data Store Read25/1 -> rampStep(oRampDataFluxMasterAngleOffset)_pitch/2
  Data Store Read18/1 -> GreaterThan4/1
  Data Store Read17/1 -> rampStep(oRampDataIdRef)_pitch/3
  Data Store Read10/1 -> GreaterThan2/1

== system Target_Control_System/Target_Control_System/MainLoop/pitchMotor_mainLoop/mainTask_pitch/motorTaskMainFastStep()/Correction Constants for Observer and Control - Pitch ==
  note: // Convert delay to angle
  note: // Now compute 1.a + 2.a:
  note: // Make the sign match the rotational direction
  note: // Add delay 3:
  note: // delay, in seconds (but the typical value will be under 100-200 us)
  note: // Delay (positive number) = np.arctan2(np.sqrt(2)*opStates->fOmegaRel_, (1-opStates->fOmegaRel_**2))
  note: // This is delay 1.b.2 MvdG: Ponder about the sign
  note: // Analytically calculate FPGA IIR filter characteristics (delay 1.b.2)
      |  // G =  1/np.sqrt(1+(fOmegaE/omega_e_3dB)**4)
  note: // Add delay 1.b.1
  note: // --- Angle and amplitude correction of the digital IIR filter ---
      | // First, we need to know the speed:
  note: // ---------------- Correction constants for observer and control ------------
      | // Sources of delay:
      | // 1. Input.
      | // a) delays from ADCs. Both voltage and current channels use identical ADCs and
      | // initial FPGA processing. The delay on the current channel is taken as a
      | // baseline.
      | //
      | // b) Extra delays in the voltage acquisition stage, due to
      | // 1) tighter analog filtering
      | // 2) the 2 pole LPF filter in the FPGA.
      | //
      | // 2. Output
      | // a) The PWM duty is updated only once per cycle, causing some delay.
      | // Additionally, the interrupt might be delayed, causing further delays.
      | //
      | // 3. User specified for testing
      | //
      | // Values of the above delays:
      | // 1.a A known constant delay is specified for each motor channel. (Mostly driven by the sinc3 filtering.
      | // Directly depends on sigma delta frequency.)
      | // 1.b.1 A known constant delay is specified for each motor channel
      | // 1.b.2 Can be calculated analytically
      | // 2.a Approximated as a constant fraction of the PWM period.
      | //
      | // Compensation order of the above delays
      | // - The entire interrupt loop runs behind reality by amount 1.a
      | // - The delay on the current acquisition is therefore not compensated at the input to the algorithm.
      | // - The voltage feedback needs to be aligned with the current feedback, and therefore needs to be
      | // corrected for delays 1.b.1 and 1.b.2. This is a phase shift applied to the voltage.
      | // - After the control loop, when the dq quantities are transformed to abc, the remaining delays are
      | // corrected by phase shifting the dq angle. These delays are 1.a, 2.a and 3.
      | //
      | // Additionally, filter 1.b.2 causes a reduction in amplitude. This is compensated too to ensure
      | // a more level flux estimate output at high speeds.
      | //
  note: // But forced angle overrules everything
  correctionConstantsObserverControl : TriggerPort  TriggerType=function-call  VariantControl=Variant
  1/sqrt(1+u^2) : Subsystem
  Abs : Abs
  Abs6 : Abs
  Abs7 : Abs  OutDataTypeStr=single
  Add12 : Sum  Inputs=|++
  Add3 : Sum  Inputs=-+
  Atan1 : Trigonometry  Operator=atan2
  Constant4 : Constant  OutDataTypeStr=single  SampleTime=-1
  Data Store Read1 : DataStoreRead  DataStoreName=oPitch  DataStoreElements=oPitch.oMot_.oState_.oRampDataOmegaERef_.fRampOut_  IndexOptions=Index vector (dialog)  Indices=1  OutputSizes=1
  Data Store Read30 : DataStoreRead  DataStoreName=oPitch  DataStoreElements=oPitch.oMot_.oParam_.fHardwareDelayCurrentAcquisition_  IndexOptions=Index vector (dialog)  Indices=1  OutputSizes=1
  Data Store Read31 : DataStoreRead  DataStoreName=oPitch  DataStoreElements=oPitch.oIsr_.oParam_.iUseSensorAngle_  IndexOptions=Index vector (dialog)  Indices=1  OutputSizes=1
  Data Store Read32 : DataStoreRead  DataStoreName=oPitch  DataStoreElements=oPitch.oMot_.oOut_.uiForcedAngle_  IndexOptions=Index vector (dialog)  Indices=1  OutputSizes=1
  Data Store Read33 : DataStoreRead  DataStoreName=oPitch  DataStoreElements=oPitch.oMot_.oParam_.fIntControlLoopDt_  IndexOptions=Index vector (dialog)  Indices=1  OutputSizes=1
  Data Store Read34 : DataStoreRead  DataStoreName=oPitch  DataStoreElements=oPitch.oMot_.oState_.oPosSensor_.fOmegaEFromSensor_  IndexOptions=Index vector (dialog)  Indices=1  OutputSizes=1
  Data Store Read35 : DataStoreRead  DataStoreName=oPitch  DataStoreElements=oPitch.oMot_.oIn_.fOmegaEObserverLpf2_  IndexOptions=Index vector (dialog)  Indices=1  OutputSizes=1
  Data Store Read36 : DataStoreRead  DataStoreName=oPitch  DataStoreElements=oPitch.oMot_.oParam_.fUphaseIirFLpfRads_  IndexOptions=Index vector (dialog)  Indices=1  OutputSizes=1
  Data Store Read38 : DataStoreRead  DataStoreName=oPitch  DataStoreElements=oPitch.oMot_.oParam_.fHardwareDelayVoltageAcquisitionExtra_  IndexOptions=Index vector (dialog)  Indices=1  OutputSizes=1
  Data Store Read39 : DataStoreRead  DataStoreName=oPitch  DataStoreElements=oPitch.oMot_.oParam_.fHardwareDelayControlLoopFraction_  IndexOptions=Index vector (dialog)  Indices=1  OutputSizes=1
  Data Store Read41 : DataStoreRead  DataStoreName=oPitch  DataStoreElements=oPitch.oMot_.oParam_.fFluxMasterAngleOffsetUser_  IndexOptions=Index vector (dialog)  Indices=1  OutputSizes=1
  Data Store Write : DataStoreWrite  DataStoreName=mdl_pitch_fOmegaE  IndexOptions=Index vector (dialog)  Indices=1  OutputSizes=1
  Data Store Write14 : DataStoreWrite  DataStoreName=oPitch  DataStoreElements=oPitch.oMot_.oState_.oRampDataFluxMasterAngleOffset_.fSetpoint_  IndexOptions=Index vector (dialog)  Indices=1  OutputSizes=1
  Data Store Write16 : DataStoreWrite  DataStoreName=oPitch  DataStoreElements=oPitch.oMot_.oState_.fOmegaRel_  IndexOptions=Index vector (dialog)  Indices=1  OutputSizes=1
  Data Store Write17 : DataStoreWrite  DataStoreName=oPitch  DataStoreElements=oPitch.oMot_.oOut_.fUphFilterAmplitudeRatio_  IndexOptions=Index vector (dialog)  Indices=1  OutputSizes=1
  Data Store Write19 : DataStoreWrite  DataStoreName=oPitch  DataStoreElements=oPitch.oMot_.oOut_.fUphFilterDelayAngleRad_  IndexOptions=Index vector (dialog)  Indices=1  OutputSizes=1
  Divide2 : Product  Inputs=/*
  Divide{4..7} (4 alike) : Product  Inputs=**
  Gain1 : Gain  Gain=sqrt(2)
  Product1 : Product
  Product2 : Product
  Saturation4 : Saturate  UpperLimit=inf  LowerLimit=0.3
  Saturation5 : Saturate  UpperLimit=pi/2  LowerLimit=-inf
  Sign2 : Signum
  Sign3 : Signum
  Sum1 : Sum  Inputs=|++
  Sum2 : Sum  Inputs=|++
  Switch6 : Switch  Criteria=u2 > Threshold
  Switch7 : Switch  Criteria=u2 > Threshold
  wires:
  Data Store Read39/1 -> Divide5/2
  Divide6/1 -> Sum2/1  "fHardwareDelayAngleRad"
  Product1/1 -> Data Store Write14/1
  Sign3/1 -> Product1/1
  Data Store Read33/1 -> Divide5/1
  Data Store Read41/1 -> Sum2/2
  Divide5/1 -> Sum1/2
  Sum2/1 -> Product1/2
  Switch7/1 -> Abs6/1, Sign2/1, Abs/1, Sign3/1, Data Store Write/1
  Sum1/1 -> Divide6/2  "fTemp"
  Data Store Read30/1 -> Sum1/1
  Abs/1 -> Divide6/1
  Add12/1 -> Saturation5/1
  Divide2/1 -> Data Store Write16/1, Divide4/1, Divide4/2, Gain1/1
  Add3/1 -> Atan1/2
  Abs7/1 -> Divide7/1
  Abs6/1 -> Product2/1, Divide2/2
  Data Store Read38/1 -> Product2/2
  Constant4/1 -> Add3/2
  Product2/1 -> Add12/2
  Atan1/1 -> Add12/1
  Data Store Read36/1 -> Divide2/1
  Saturation4/1 -> Data Store Write17/1
  Divide4/1 -> 1/sqrt(1+u^2)/1(fTemp), Add3/1  "fTemp"
  Divide7/1 -> Data Store Write19/1
  Gain1/1 -> Atan1/1
  Saturation5/1 -> Abs7/1
  1/sqrt(1+u^2)/1(Out1) -> Saturation4/1
  Sign2/1 -> Divide7/2
  Data Store Read1/1 -> Switch7/1
  Data Store Read32/1 -> Switch7/2
  Switch6/1 -> Switch7/3
  Data Store Read35/1 -> Switch6/3
  Data Store Read34/1 -> Switch6/1
  Data Store Read31/1 -> Switch6/2
